simulink model "Copy_of_controlled"  (Simulink 8.9)
settings: Solver=ode45  StartTime=0.0  StopTime=20  MaxStep=1e-4  RelTol=1e-6  EnableMultiTasking=on
undefined symbols (not defined in the file or in its folder): DiscIntNeverNeededParam, jointObj
libraries: simulink x3, cjt_library_controllers x2, cjt_library_models x1, cstblocks x1, cjt_library_observers x1
settings Model: SuppressorTable=22 serialization::archive 11 0 6 0 0 0 11 0  Creator=wesley  LastModifiedBy=wesley
settings DataIOCC: SignalLoggingSaveFormat=Dataset
settings DebuggingCC: SolverPrmCheckMsg=warning  FcnCallInpInsideContextMsg=error  AllowSymbolicDim=off  StateNameClashWarn=none
settings GRTTargetCC: CombineOutputUpdateFcns=on  GRTInterface=off

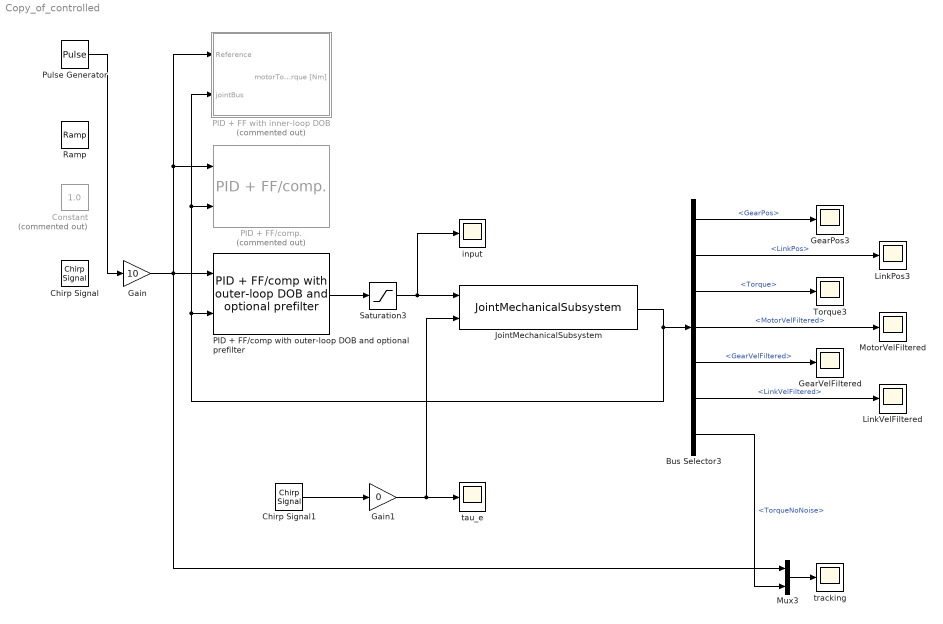
== system Copy_of_controlled ==
  Bus Selector3 : BusSelector  OutputSignals=GearPos,LinkPos,Torque,MotorVelFiltered,GearVelFiltered,LinkVelFiltered,TorqueNoNoise
  Chirp Signal : simulink/Sources/Chirp Signal  f1=0.1  T=120  f2=120
  Chirp Signal1 : simulink/Sources/Chirp Signal  f1=0.1  T=120  f2=120
  Constant : Constant  Commented=on  Value=1.0
  Gain : Gain  Gain=10
  Gain1 : Gain  Gain=0
  GearPos3 : Scope
  GearVelFiltered : Scope
  JointMechanicalSubsystem : cjt_library_models/Joint models/JointMechanicalSubsystem  jointObj=jointObj  fc_vel=1e3  fc_torque=1e3  input_delay=0  output_delay=1  quantize=on  quantize_bits=19  input_noise_enabled=on  output_noise_enabled=on  var_u=0.12^2  var_y=1.8e-10
  LinkPos3 : Scope
  LinkVelFiltered : Scope
  MotorVelFiltered : Scope
  Mux3 : Mux  Inputs=2
  PID + FF with inner-loop DOB : Subsystem  Commented=on  AncestorBlock=cjt_library_controllers/Controllers/PID + FF with inner-loop DOB  mask(PID + FF with inner-loop DOB){jointObj=jointObj, Kp=1, Ki=0, Kd=0.01, N=2*pi*1000, derivative_select=Output, ff_comp_switch=Feed-forward, DOB_enabled=off, f_c=20, measIdx=[7], DOB_order=0}
      mask prompts: jointObj "Joint Object"; Kp "Proportional gain Kp"; Ki "Integral gain Ki"; Kd "Derivative gain Kd"; N "Derivative filter coefficient N"; derivative_select "Derivative action on:"; ff_comp_switch "Spring force rejection"; DOB_enabled "DOB enabled"; f_c "DOB cut-off frequency [Hz]"; measIdx "Measurement index"; DOB_order "DOB order (0 = auto minimum order)"
      mask help:
      | This block implements a PID torque controller with optional feed-forward or compensation term, supplemented with an inner-loop DOB.
      |
      | Click >Help< for further documentation.
      mask init:
      | % Get linear dynamics matrices
      | [A, B, C, D, I, R, K] = jointObj.getDynamicsMatrices();
      mask Help:
      | This block implements a PID torque controller with optional feed-forward or compensation term, supplemented with an inner-loop DOB. The DOB is based on the nominal open-loop plant dynamics.
      | 
      | <b>Mask parameters:</b>
      | 
      | Joint Object: The class name of the CJT joint class name or the variable representing an instance of a CJT joint class.
      | K<sub>P</sub>, K<sub>I</sub>, K<sub>D</sub>: Proportional, derivative, and integral gain, respectively.
      | N: Derivative low-pass filter coefficient
      | DOB cutoff frequency: Cut-off frequency computed for the low-pass filter that must be used to make the inverse transfer function realisible.
      | Measurement index: Measured plant output that should be used for the DOB.
      | 
      | 
      | <b>References:</b>
      | 
      | H. S. Lee and M. Tomizuka, "Robust motion controller design for high-accuracy positioning systems". In IEEE Transactions on Industrial Electronics, vol. 43, no. 1, pp. 48--55, 1996.
      | 
      | W. Roozing, J. Malzahn, D. G. Caldwell, and N. G. Tsagarakis, "Comparison of open-loop and closed-loop disturbance observers for series elastic actuators". In Intelligent Robots and Systems (IROS), 2016 IEEE/RSJ International Conference on, 2016, pp. 3842--3847.
      | 
      | M. C. Readman, Flexible Joint Robots. CRC press, 1994.
      mask TypeOptions derivative_select: Error | Output
      mask TypeOptions ff_comp_switch: Compensation | Feed-forward | Off
      mask Callback DOB_enabled:
      | % Toggle all DOB fields
      | fields = {  'f_c', ...
      |             'measIdx', ...
      |             'DOB_order', ...
      |          };
      | toggleMaskFields(gcbh, 'DOB_enabled', fields, 'on');
      mask DialogControl Container3 Prompt: Controller
      mask DialogControl ParameterGroupVar Prompt: DOB parameters
  PID + FF/comp with outer-loop DOB and optional prefilter : cjt_library_controllers/Controllers/PID + FF//comp with outer-loop DOB and optional prefilter  jointObj=jointObj  Kp=1  Ki=0  Kd=0.01  N=2*pi*1000  derivative_select=Output  ff_comp_switch=Feed-forward  DOB_enable_switch=On  premult_enable_switch=Off  loadData=off  modelFname=DOB_results.mat  f_c_FF=20  f_c_DOB=30  DOB_order=0
  PID + FF/comp. : cjt_library_controllers/Controllers/PID + FF//comp.  Commented=on  jointObj=jointObj  Kp=1  Ki=0  Kd=0.01  N=2*pi*1000  derivative_select=Output  ff_comp_switch=Feed-forward
  Pulse Generator : DiscretePulseGenerator  PulseType=Time based  Amplitude=4  Period=5  PulseWidth=50
  Ramp : simulink/Sources/Ramp  slope=0.3  start=1  X0=0
  Saturation3 : Saturate  UpperLimit=inf  LowerLimit=-inf
  Torque3 : Scope
  input : Scope
  tau_e : Scope
  tracking : Scope
  wires:
  Pulse Generator/1 -> Gain/1
  Bus Selector3/2 -> LinkPos3/1  "<LinkPos>"
  Bus Selector3/3 -> Torque3/1  "<Torque>"
  Mux3/1 -> tracking/1
  Bus Selector3/1 -> GearPos3/1  "<GearPos>"
  JointMechanicalSubsystem/1 -> PID + FF with inner-loop DOB/2(jointBus), PID + FF/comp./2, PID + FF/comp with outer-loop DOB and optional prefilter/2, Bus Selector3/1
  PID + FF/comp with outer-loop DOB and optional prefilter/1 -> Saturation3/1
  Saturation3/1 -> JointMechanicalSubsystem/1, input/1
  Gain/1 -> PID + FF with inner-loop DOB/1(Reference), PID + FF/comp./1, PID + FF/comp with outer-loop DOB and optional prefilter/1, Mux3/1
  Gain1/1 -> JointMechanicalSubsystem/2, tau_e/1
  Chirp Signal1/1 -> Gain1/1
  Bus Selector3/4 -> MotorVelFiltered/1  "<MotorVelFiltered>"
  Bus Selector3/5 -> GearVelFiltered/1  "<GearVelFiltered>"
  Bus Selector3/6 -> LinkVelFiltered/1  "<LinkVelFiltered>"
  Bus Selector3/7 -> Mux3/2  "<TorqueNoNoise>"

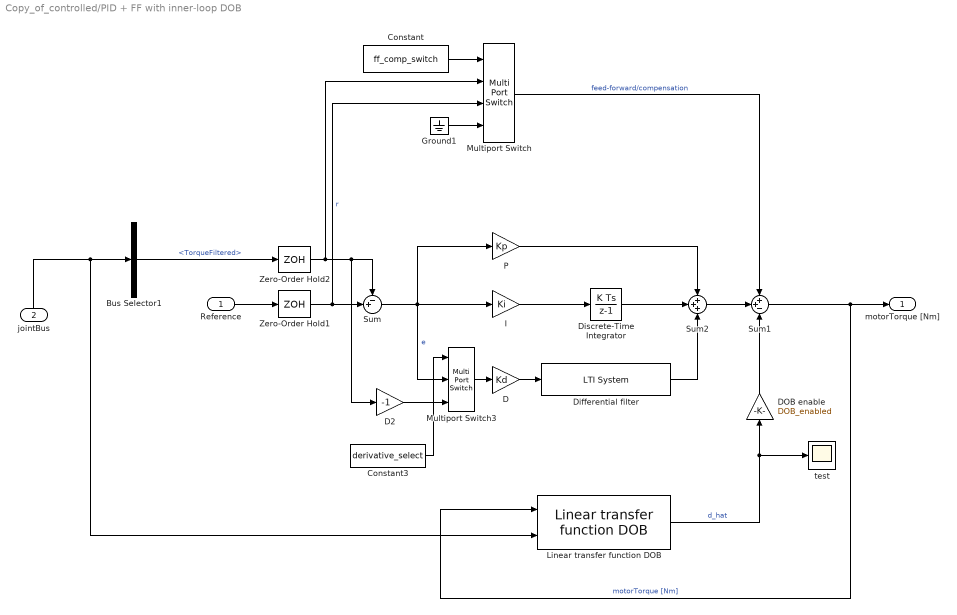
== system Copy_of_controlled/PID + FF with inner-loop DOB ==
  Reference : Inport
  jointBus : Inport  Port=2
  Bus Selector1 : BusSelector  OutputSignals=TorqueFiltered
  Constant : Constant  Value=ff_comp_switch
  Constant3 : Constant  Value=derivative_select
  D : Gain  Gain=Kd
  D2 : Gain  Gain=-1
  DOB enable : Gain  Gain=DOB_enabled
  Differential filter : cstblocks/LTI System  sys=c2d(tf([N 0], [1, N]), jointObj.Ts, 'tustin')  IC=[]
  Discrete-Time Integrator : DiscreteIntegrator  SampleTime=-1  ICPrevOutput=DiscIntNeverNeededParam  ICPrevScaledInput=DiscIntNeverNeededParam
  Ground1 : Ground
  I : Gain  Gain=Ki
  Linear transfer function DOB : cjt_library_observers/Observers/Linear transfer function DOB  loadData=off  modelFname=DOB_results.mat  jointObj=jointObj  f_c=f_c  measIdx=measIdx  DOB_order=DOB_order
  Multiport Switch : MultiPortSwitch
  Multiport Switch3 : MultiPortSwitch  Inputs=2
  P : Gain  Gain=Kp
  Sum : Sum  Inputs=-+|
  Sum1 : Sum  Inputs=++-
  Sum2 : Sum  Inputs=+++
  Zero-Order Hold1 : ZeroOrderHold  SampleTime=jointObj.Ts
  Zero-Order Hold2 : ZeroOrderHold  SampleTime=jointObj.Ts
  test : Scope
  motorTorque [Nm] : Outport
  wires:
  Multiport Switch3/1 -> D/1
  Sum/1 -> Multiport Switch3/2, P/1, I/1  "e"
  Constant3/1 -> Multiport Switch3/1
  D2/1 -> Multiport Switch3/3
  Zero-Order Hold2/1 -> Multiport Switch/2, Sum/1, D2/1
  DOB enable/1 -> Sum1/3
  Sum2/1 -> Sum1/2
  Differential filter/1 -> Sum2/3
  P/1 -> Sum2/1
  Discrete-Time Integrator/1 -> Sum2/2
  I/1 -> Discrete-Time Integrator/1
  D/1 -> Differential filter/1
  Linear transfer function DOB/1 -> test/1, DOB enable/1  "d_hat"
  jointBus/1 -> Bus Selector1/1, Linear transfer function DOB/2
  Bus Selector1/1 -> Zero-Order Hold2/1  "<TorqueFiltered>"
  Sum1/1 -> motorTorque [Nm]/1, Linear transfer function DOB/1  "motorTorque [Nm]"
  Reference/1 -> Zero-Order Hold1/1
  Multiport Switch/1 -> Sum1/1  "feed-forward/compensation"
  Constant/1 -> Multiport Switch/1
  Ground1/1 -> Multiport Switch/4
  Zero-Order Hold1/1 -> Multiport Switch/3, Sum/2  "r"

== matlab function JointMechanicalSubsystem/nonLinDynamicsFcn ==
  data: tau output double; x input double; y output double
function [tau, y] = nonLinDynamics(x)
%#codegen

params.a_CU = 0.003900;
params.c_CU = 380.000000;
params.c_FE = 460.000000;
params.diam = 93.000000;
params.len = 163.000000;
params.m = 1.000000;
params.I_m = 0.230000;
params.I_g = 0.071700;
params.I_l = 0.000100;
params.k_g = 16000.000000;
params.k_b = 6000.000000;
params.d_m = 0.003600;
params.d_g = 2.200000;
params.d_l = 0.000000;
params.d_m_n = 0.003600;
params.d_g_n = 2.200000;
params.d_l_n = 0.000000;
params.d_mg = 100.000000;
params.d_gl = 0.000000;
params.d_cm = 2.640000;
params.d_cg = 3.280000;
params.d_cl = 0.000000;
params.d_cm_n = 2.640000;
params.d_cg_n = 3.280000;
params.d_cl_n = 0.000000;
params.d_s = 0.000000;
params.v_s = 0.000000;
params.rip_types = [];
params.rip_a1 = [];
params.rip_a2 = [];
params.rip_f = [];
params.n = 80.000000;
params.k_t = 0.078000;
params.r = 0.318000;
params.x = 0.000200;
params.p = 6.000000;
params.v_0 = 48.000000;
params.i_p = 30.000000;
params.dq_p = 7.728400;
params.r_th1 = 3.136400;
params.r_th2 = 32.663700;
params.T_thw = 98.081700;
params.T_thm = 4679.965500;
params.Tmp_WMax = 155.000000;
params.Tmp_ANom = 25.000000;
params.name = 'cjt_Orange_80_6000_output_fixed_rigid_gearbox';
params.paramName = 'cjt_Orange_80_6000';
params.modelName = 'output_fixed_rigid_gearbox';
params.nonlinearModelName = '';
params.electricalModelName = 'electric_dyn_zero_inductance';
params.Ts = 0.001000;
params.Ts_elec = 0.000100;
tau = zeros(3,1);
y = zeros(7,1);
	end
